simulink model "hydrofoil_sim_unified"  (R2024b)
settings: Solver=VariableStepAuto  StartTime=0.0  StopTime=20  FixedStep=0.05  MaxStep=0.2  RelTol=1e-3
values from neighbouring files (symbols this model uses):
  AfoilA = 0.046    [model_parameters.m]
  AfoilFP = 0.048    [model_parameters.m]
  AfoilFS = 0.048    [model_parameters.m]
  alpha0012 = data0012(:,1)    [model_parameters.m]
  alpha63412wing = data63412wing(:,1)    [model_parameters.m]
  cd0012 = data0012(:,3)    [model_parameters.m]
  cdi63412wing = data63412wing(:,4)    [model_parameters.m]
  cdv63412wing = data63412wing(:,5)    [model_parameters.m]
  cl63412wing = data63412wing(:,3)    [model_parameters.m]
  cm63412wing = data63412wing(:,9)    [model_parameters.m]
  csA = 0.1    [model_parameters.m]
  csF = 0.08    [model_parameters.m]
  deltat = 1/100    (= 0.01)    [model_parameters.m]
  foilA_ARM = [-dxa, dya, dza]    [model_parameters.m]
  foilFP_ARM = [dxf, -dyf, dzf]    [model_parameters.m]
  foilFS_ARM = [dxf, dyf, dzf]    [model_parameters.m]
  g = 9.81    [model_parameters.m]
  LAd = 0.08*pi*(0.8)^3/64    (= 0.0020106192983)    [model_parameters.m]
  LFPd = integral(fpint, foilFP_ARM(2)-0.4, foilFP_ARM(2)+0.4)    [model_parameters.m]
  LFSd = integral(fsint, foilFS_ARM(2)-0.4, foilFS_ARM(2)+0.4)    [model_parameters.m]
  M_RB_1 = inv(M_RB)    [dimensionalize_model.m]    (also in model_parameters.m = M_RB^(-1))
  MAC_A = 0.08    [model_parameters.m]
  MAC_FP = 0.08    [model_parameters.m]
  MAC_FS = 0.08    [model_parameters.m]
  mass = 215    [dimensionalize_model.m]    (also in model_parameters.m)
  propwake = 0.05    [model_parameters.m]
  psd_acc = (9.81*60*1e-6)^2    (= 3.4644996e-07)    [model_parameters.m]
  psd_gyro = (1.222*1e-4)^2    (= 1.493284e-08)    [model_parameters.m]
  r_g = [0; 0; 0]    [dimensionalize_model.m]    (also in model_parameters.m = [xg, yg, zg])
  rho = 1024.8    [model_parameters.m]
  seed_accX = 1324    [model_parameters.m]
  seed_accZ = 1432    [model_parameters.m]
  seed_gps = 4321    [model_parameters.m]
  seed_gyroX = 243251    [model_parameters.m]
  seed_gyroY = 3124234    [model_parameters.m]
  seed_pitch = 7568    [model_parameters.m]
  seed_roll = 35642    [model_parameters.m]
  seed_sonar = 1234    [model_parameters.m]
  setpoint_signals = setpoints.preview    [model_parameters.m]
  sonar_position = [dxf+0.5; 0; -0.1]    [model_parameters.m]
  spanA = 0.76    [model_parameters.m]
  spanFP = 0.76    [model_parameters.m]
  spanFS = 0.76    [model_parameters.m]
  tA = 0.12*0.08    (= 0.0096)    [model_parameters.m]
  tFP = 0.12*0.08    (= 0.0096)    [model_parameters.m]
  tFS = 0.12*0.08    (= 0.0096)    [model_parameters.m]
  usted = 7    [model_parameters.m]
  var_angle = deg2rad(0.2)^2    [model_parameters.m]
  var_gps = 0.05^2    (= 0.0025)    [model_parameters.m]
  var_sonar = 0.002^2    (= 4e-06)    [model_parameters.m]
  wagC1 = 0.165    [model_parameters.m]
  wagC2 = 0.335    [model_parameters.m]
  wage1 = 0.0455*(usted/(MAC_FP/2))    (= 7.9625)    [model_parameters.m]
  wage2 = 0.3*(usted/(MAC_FP/2))    (= 52.5)    [model_parameters.m]
  wave_data = struct('amplitude',0,'omega',0,'wavenumber',0,'phase',0,'direction',0)    [model_parameters.m]
  zpr = dza    (= 0.96)    [model_parameters.m]
undefined symbols (not defined in the file or in its folder): act_lims, actuation_tau, bA, bB, bC, bD, dLTI_array_IDP, dLTI_array_IP, Ka, Klqid, magnitude, PredictionHorizon, set, Ts_reference_preview, V_vals
libraries: mssSimulink x15, mpclib x10, simulink x6, simulink_extras x5, cstblocks x4, matrix_library x3, slpidlib x1
(part 1 of 3)
settings Model: SimulationMode=accelerator  PauseTimes=0.5  SnapshotInterval=1  Creator=jskounakis  LastModifiedBy=jskounakis
settings DataIOCC: ExternalInput=setpoint_reference  InitialState=getstatestruct(report6)
settings OptimizationCC: ReuseModelBlockBuffer=off
settings RTWCC: GPUComputeCapability=3.5

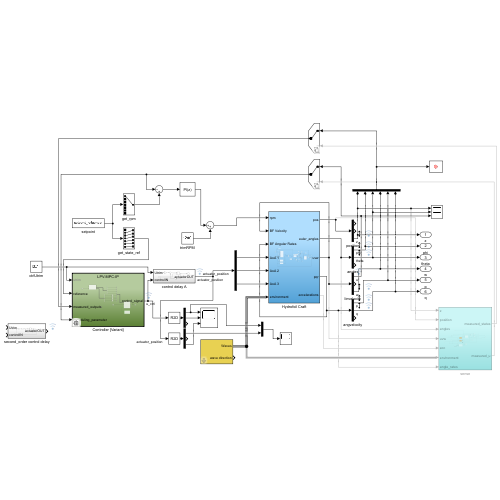
[thumbnail: Simulink's stored preview of the top-level diagram]
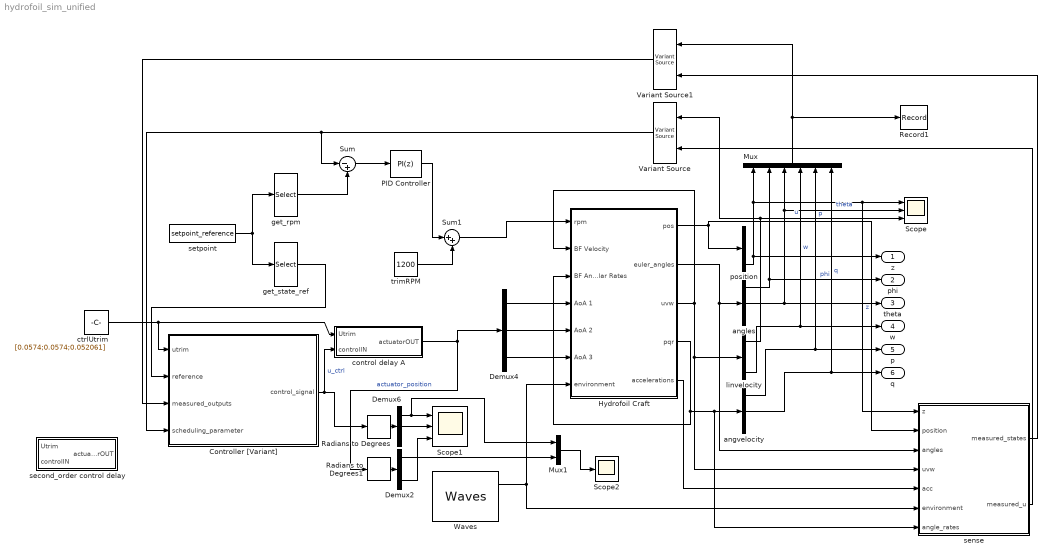
== system hydrofoil_sim_unified ==
  Controller [Variant] : Subsystem  Variant=on  VariantActivationTime=startup
  Demux2 : Demux  Outputs=3
  Demux4 : Demux  Outputs=3
  Demux6 : Demux  Outputs=3
  Hydrofoil Craft : Subsystem
  Mux : Mux  Inputs=6
  Mux1 : Mux  Inputs=2
  PID Controller : slpidlib/PID Controller  Controller=PI  Form=Parallel  TimeDomain=Discrete-time  UseExternalTs=off  SampleTime=1/100  IntegratorMethod=Forward Euler  FilterMethod=Forward Euler  ControllerParametersSource=internal  P=250  I=200  UseKiTs=off  D=0  UseExternalDerivativeSource=off  N=100  UseFilter=on  TunerSelectOption=Transfer Function Based (PID Tuner App)  InitialConditionSource=internal  InitialConditionForIntegrator=0  InitialConditionForFilter=0  DifferentiatorICPrevScaledInput=0  ExternalReset=none  TrackingMode=off  Kt=1  LimitOutput=off  SatLimitsSource=internal  UpperSaturationLimit=inf  LowerSaturationLimit=-inf  LinearizeAsGain=on  AntiWindupMode=none  Kb=1  LimitIntegrator=off  UpperIntegratorSaturationLimit=inf  LowerIntegratorSaturationLimit=-inf  POutMin=[]  POutMax=[]  IOutMin=[]  IOutMax=[]  DOutMin=[]  DOutMax=[]  NOutMin=[]  NOutMax=[]  SumOutMin=[]  SumOutMax=[]  SaturationOutMin=[]  SaturationOutMax=[]  PParamMin=[]  PParamMax=[]  IParamMin=[]  IParamMax=[]  DParamMin=[]  DParamMax=[]  NParamMin=[]  NParamMax=[]  KbParamMin=[]  KbParamMax=[]  KtParamMin=[]  KtParamMax=[]  KbOutMin=[]  KbOutMax=[]  KtOutMin=[]  KtOutMax=[]  IntegratorOutMin=[]  IntegratorOutMax=[]  FilterOutMin=[]  FilterOutMax=[]  SumI1OutMin=[]  SumI1OutMax=[]  SumI2OutMin=[]  SumI2OutMax=[]  SumI3OutMin=[]  SumI3OutMax=[]  SumI4OutMin=[]  SumI4OutMax=[]  SumDOutMin=[]  SumDOutMax=[]  DifferentiatorOutMin=[]  DifferentiatorOutMax=[]  FilterDiffOutCoefMin=[]  FilterDiffOutCoefMax=[]  ReciprocalOutMin=[]  ReciprocalOutMax=[]  SumDenOutMin=[]  SumDenOutMax=[]  SumNumOutMin=[]  SumNumOutMax=[]  DivideOutMin=[]  DivideOutMax=[]  UdiffTsProdOutMin=[]  UdiffTsProdOutMax=[]  NTsProdOutMin=[]  NTsProdOutMax=[]  UintegralTsProdOutMin=[]  UintegralTsProdOutMax=[]  UngainTsProdOutMin=[]  UngainTsProdOutMax=[]  ClampingZeroOutDataTypeStr=Inherit: Inherit via back propagation  ClampingZeroOutMin=[]  ClampingZeroOutMax=[]  FilterDenConstantOutDataTypeStr=Inherit: Inherit via back propagation  FilterDenConstantOutMin=[]  FilterDenConstantOutMax=[]  PCopyOutDataTypeStr=Inherit: Inherit via back propagation  PCopyOutMin=[]  PCopyOutMax=[]  NCopyOutDataTypeStr=Inherit: Inherit via back propagation  NCopyOutMin=[]  NCopyOutMax=[]  IntegratorContinuousStateAttributes=''  IntegratorStateMustResolveToSignalObject=off  IntegratorRTWStateStorageClass=Auto  FilterContinuousStateAttributes=''  FilterStateMustResolveToSignalObject=off  FilterRTWStateStorageClass=Auto  ParallelPVariant=InternalParameters  IdealPVariant=Disabled  IVariant=InternalParameters  DVariant=Disabled  IntegratorVariant=Discrete  SatVariant=Disabled  AWVariant=Passthrough  PCopyVariant=Disabled  TRVariant=Disabled  FdbkBlocksVariant=Forward  IdealPFdbkVariant=Disabled  SatFdbkVariant=Disabled  DerivativeFilterVariant=Disabled  NVariant=Disabled  NCopyVariant=Disabled_SignalSpec  FilterICVariant=Disabled  IntegratorICVariant=InternalICs  ExternalResetVariant=Disabled  TRSumVariant=Passthrough  SumFdbkVariant=Disabled  SumVariant=Sum_PI  TsampFilterVariant=InternalTs  TsampNgainVariant=Passthrough  TsampIntegralVariant=Disabled_SignalSpec  ExternalSaturationOutDataTypeStr=Inherit: Same as second input  DerivativeSourceVariant=Disabled  PreIntVariant=InternalPreInt
  Radians to Degrees : simulink_extras/Transformations/Radians to Degrees
  Radians to Degrees1 : simulink_extras/Transformations/Radians to Degrees
  Record1 : Record  FileSettingsInternal="{\"entries\":[{\"content\":{\"excelSettings\":{\"content\":{},\"type\":\"Streamout.ExcelSettings\"}},\"type\":\"Streamout.FileSettingStorage\",\"uuid\":\"\"}],\"packageUris\":[\"http:\\/\\/schema.mathworks.com\\/mf0\\/streamout_blocks\\/R2020a\"],\"version\":\"1.0\"}"  Layout=[1 1]  SignalsInternal="{\"entries\":[{\"content\":{\"signals\":[{\"content\":{\"blockPath\":[],\"dimensions\":[6],\"domain\":\"\",\"hasChildren\":true,\"lineColor\":\"#7e2f8e\",\"lineWidth\":2,\"port\":1,\"sid\":[\"\"],\"signalID\":1,\"signalName\":\"Mux\"},\"type\":\"RecordBlkView.Signal\",\"uuid\":\"\"},{\"content\":{\"blockPath\":[],\"channel\":[1],\"dimensions\":[6],\"domain\":\"\",\"lineColor\":\"#ff6929\",\"lineWidth\":2,\"parentID\":1,\"plots\":[ 1, 27 ],\"port\":1,\"sid\":[\"\"],\"signalID\":2,\"signalName\":\"Mux\"},\"type\":\"RecordBlkView.Signal\",\"uuid\":\"\"},{\"content\":{\"blockPath\":[],\"channel\":[2],\"dimensions\":[6],\"domain\":\"\",\"lineColor\":\"#b746ff\",\"lineWidth\":2,\"parentID\":1,\"plots\":[ 1 ],\"port\":1,\"sid\":[\"\"],\"signalID\":3,\"signalName\":\"Mux\"},\"type\":\"RecordBlkView.Signal\",\"uuid\":\"\"},{\"content\":{\"blockPath\":[],\"channel\":[3],\"dimensions\":[6],\"domain\":\"\",\"lineColor\":\"#64d413\",\"lineWidth\":2,\"parentID\":1,\"plots\":[ 1, 27 ],\"port\":1,\"sid\":[\"\"],\"signalID\":4,\"signalName\":\"Mux\"},\"type\":\"RecordBlkView.Signal\",\"uuid\":\"\"},{\"content\":{\"blockPath\":[],\"channel\":[4],\"dimensions\":[6],\"domain\":\"\",\"lineColor\":\"#ff13a6\",\"lineWidth\":2,\"parentID\":1,\"plots\":[ 1 ],\"port\":1,\"sid\":[\"\"],\"signalID\":5,\"signalName\":\"Mux\"},\"type\":\"RecordBlkView.Signal\",\"uuid\":\"\"},{\"content\":{\"blockPath\":[],\"channel\":[5],\"dimensions\":[6],\"domain\":\"\",\"lineColor\":\"#ff6929\",\"lineWidth\":2,\"parentID\":1,\"plots\":[ 1 ],\"port\":1,\"sid\":[\"\"],\"signalID\":6,\"signalName\":\"Mux\"},\"type\":\"RecordBlkView.Signal\",\"uuid\":\"\"},{\"content\":{\"blockPath\":[],\"channel\":[6],\"dimensions\":[6],\"domain\":\"\",\"lineColor\":\"#139fff\",\"lineWidth\":2,\"parentID\":1,\"plots\":[ 1 ],\"port\":1,\"sid\":[\"\"],\"signalID\":7,\"signalName\":\"Mux\"},\"type\":\"RecordBlkView.Signal\",\"uuid\":\"\"}]},\"type\":\"RecordBlkView.InputSignals\",\"uuid\":\"\"}],\"packageUris\":[\"http:\\/\\/schema.mathworks.com\\/mf0\\/streamout_blocks\\/R2020a\"],\"version\":\"1.0\"}"  VisualizationBindings="{\"sparklinesplugin\":{\"info\":[{\"bindingParametersList\":[],\"subplotID\":1}]}}"
  Scope : Scope  NumInputPorts=3
  Scope1 : Scope  NumInputPorts=3
  Scope2 : Scope
  Sum : Sum  Inputs=|-+
  Sum1 : Sum  Inputs=|++
  Variant Source : VariantSource
  Variant Source1 : VariantSource
  Waves : mssSimulink/Environment/Waves/Waves  spectrum_type=Predefined waves  disp_flag=off  plot_spectrum=off  plot_realization=off  hs=0.4  omega_peak=6  psi_mean=pi  gamma=3.3  spread=3  depth=inf  nfreq=40  ndir=10  energylim=40  freq_cutoff=2  dir_cutoff=pi/8  rand_seed=seed_waves  rand_freq=on  rand_dir=on  Zeta_a=wave_data.amplitude  Omega=wave_data.omega  Phase=wave_data.phase  Wavenum=wave_data.wavenumber  Psi=wave_data.direction
  angles : Demux  Outputs=3
  angvelocity : Demux  Outputs=3
  control delay A : Subsystem
  ctrlUtrim : Constant  Value=[0.0574;0.0574;0.052061]
  get_rpm : Selector  InputPortWidth=7  IndexOptions=Index vector (dialog)  Indices=[1]  OutputSizes=1
  get_state_ref : Selector  InputPortWidth=7  IndexOptions=Index vector (dialog)  Indices=[2:7]  OutputSizes=1
  linvelocity : Demux  Outputs=3
  position : Demux  Outputs=3
  second_order control delay : Subsystem
  sense : Subsystem
  setpoint : FromWorkspace  VariableName=setpoint_reference
  trimRPM : Constant  Value=1200
  z : Outport
  phi : Outport  Port=2
  theta : Outport  Port=3
  w : Outport  Port=4
  p : Outport  Port=5
  q : Outport  Port=6
  wires:
  ctrlUtrim/1 -> control delay A/1(Utrim), Controller [Variant]/1(utrim)
  Demux4/1 -> Hydrofoil Craft/4(AoA 1)
  Demux4/2 -> Hydrofoil Craft/5(AoA 2)
  Controller [Variant]/1(control_signal) -> control delay A/2(controlIN), Radians to Degrees/1  "u_ctrl"
  angvelocity/2 -> Mux/6, q/1  "q"
  Hydrofoil Craft/4(pqr) -> angvelocity/1, sense/7(angle_rates), Hydrofoil Craft/3(BF Angular Rates)
  Mux/1 -> Variant Source1/1, Record1/1
  angvelocity/1 -> Mux/5, p/1  "p"
  Hydrofoil Craft/3(uvw) -> sense/4(uvw), linvelocity/1, Hydrofoil Craft/2(BF Velocity)
  Hydrofoil Craft/2(euler_angles) -> sense/3(angles), angles/1
  linvelocity/3 -> Mux/4, w/1  "w"
  angles/1 -> Mux/2, phi/1  "phi"
  Hydrofoil Craft/1(pos) -> position/1, sense/2(position)
  angles/2 -> theta/1, Mux/3, Scope/2  "theta"
  position/3 -> Mux/1, Scope/1, sense/1(z), z/1  "z"
  Demux4/3 -> Hydrofoil Craft/6(AoA 3)
  linvelocity/1 -> Variant Source/1, Scope/3  "u"
  Radians to Degrees/1 -> Demux6/1
  Radians to Degrees1/1 -> Demux2/1
  setpoint/1 -> get_rpm/1, get_state_ref/1
  get_state_ref/1 -> Controller [Variant]/2(reference)
  Waves/1 -> sense/6(environment), Hydrofoil Craft/7(environment)
  Demux6/1 -> Mux1/1, Scope1/1
  Demux6/2 -> Scope1/2
  Hydrofoil Craft/5(accelerations) -> sense/5(acc)
  sense/1(measured_states) -> Variant Source1/2
  sense/2(measured_u) -> Variant Source/2
  Variant Source1/1 -> Controller [Variant]/3(measured_outputs)
  Variant Source/1 -> Sum/1, Controller [Variant]/4(scheduling_parameter)
  Mux1/1 -> Scope2/1
  Demux2/1 -> Mux1/2
  control delay A/1(actuatorOUT) -> Demux4/1, Radians to Degrees1/1  "actuator_position"
  Demux2/3 -> Scope1/3
  Sum/1 -> PID Controller/1
  trimRPM/1 -> Sum1/2
  PID Controller/1 -> Sum1/1
  get_rpm/1 -> Sum/2
  Sum1/1 -> Hydrofoil Craft/1(rpm)

== system hydrofoil_sim_unified/Controller [Variant] ==
  note: LPV-MPC
  note: MPC
  note: LQI
  note: 1) Add Subsystem or Model blocks as valid variant choices.
      | 2) You cannot connect blocks at this level. At simulation, connectivity is automatically
      | determined, based on the active variant and port name matching.
  utrim : Inport
  reference : Inport  Port=2
  measured_outputs : Inport  Port=3
  scheduling_parameter : Inport  Port=4
  LPV-MPC-IDP : Subsystem  TreatAsAtomicUnit=on  VariantControl=control_flag == 12
  LPV-MPC-IP : Subsystem  TreatAsAtomicUnit=on  VariantControl=control_flag == 11
  LQI : Subsystem  TreatAsAtomicUnit=on  VariantControl=control_flag == 1
  LQI-S : Subsystem  TreatAsAtomicUnit=on  VariantControl=control_flag == 2
  LQI-SW : Subsystem  TreatAsAtomicUnit=on  VariantControl=control_flag == 3
  MPC : Subsystem  TreatAsAtomicUnit=on  VariantControl=control_flag == 4
  MPC-I : Subsystem  TreatAsAtomicUnit=on  VariantControl=control_flag == 5
  MPC-ID : Subsystem  TreatAsAtomicUnit=on  VariantControl=control_flag == 8
  MPC-IDP : Subsystem  TreatAsAtomicUnit=on  VariantControl=control_flag == 10
  MPC-IO : Subsystem  TreatAsAtomicUnit=on  VariantControl=control_flag == 7
  MPC-IOP : Subsystem  TreatAsAtomicUnit=on  VariantControl=control_flag == 13
  MPC-IP : Subsystem  TreatAsAtomicUnit=on  VariantControl=control_flag == 9
  MPC-O : Subsystem  TreatAsAtomicUnit=on  VariantControl=control_flag == 6
  control_signal : Outport

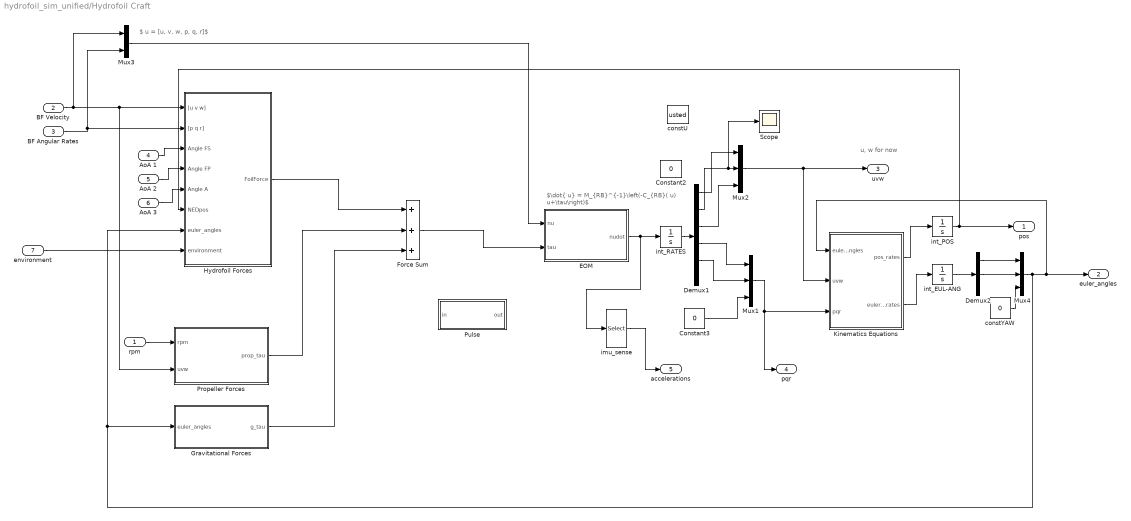
== system hydrofoil_sim_unified/Hydrofoil Craft ==
  note: $\nu = [u, v, w, p, q, r]$
  note: $\dot{\nu} = M_{RB}^{-1}\left(-C_{RB}(\nu)\nu+\tau\right)$
  note: u, w for now
  rpm : Inport
  BF Velocity : Inport  Port=2
  BF Angular Rates : Inport  Port=3
  AoA 1 : Inport  Port=4
  AoA 2 : Inport  Port=5
  AoA 3 : Inport  Port=6
  environment : Inport  Port=7
  Constant2 : Constant  Value=0
  Constant3 : Constant  Value=0
  Demux1 : Demux  Outputs=6
  Demux2 : Demux  Outputs=3
  EOM : Subsystem
  Force Sum : Sum  Inputs=+++
  Gravitational Forces : MATLAB Function  TreatAsAtomicUnit=on
  Hydrofoil Forces : Subsystem
  Kinematics Equations : MATLAB Function  TreatAsAtomicUnit=on
  Mux1 : Mux  Inputs=3
  Mux2 : Mux  Inputs=3
  Mux3 : Mux  Inputs=2
  Mux4 : Mux  Inputs=3
  Propeller Forces : Subsystem
  Pulse : Subsystem
  Scope : Scope
  constU : Constant  Value=usted
  constYAW : Constant  Value=0
  imu_sense : Selector  InputPortWidth=6  IndexOptions=Index vector (dialog)  Indices=[1:3]  OutputSizes=1
  int_EUL-ANG : Integrator  InitialCondition=[0;0;0]
  int_POS : Integrator  InitialCondition=[0;0;-0.3]
  int_RATES : Integrator  InitialCondition=[7;0;0;0;0;0]
  pos : Outport
  euler_angles : Outport  Port=2
  uvw : Outport  Port=3
  pqr : Outport  Port=4
  accelerations : Outport  Port=5
  wires:
  BF Angular Rates/1 -> Mux3/2, Hydrofoil Forces/2("[p q r]")
  BF Velocity/1 -> Mux3/1, Propeller Forces/2(uvw), Hydrofoil Forces/1("[u v w]")
  int_RATES/1 -> Demux1/1
  Mux1/1 -> Kinematics Equations/3(pqr), pqr/1
  Demux1/3 -> Mux2/3
  Demux1/5 -> Mux1/2
  Mux2/1 -> Kinematics Equations/2(uvw), uvw/1
  Kinematics Equations/1(pos_rates) -> int_POS/1
  AoA 2/1 -> Hydrofoil Forces/4(Angle FP)
  AoA 3/1 -> Hydrofoil Forces/5(Angle A)
  AoA 1/1 -> Hydrofoil Forces/3(Angle FS)
  Demux2/1 -> Mux4/1
  Demux2/2 -> Mux4/2
  Mux4/1 -> Hydrofoil Forces/7(euler_angles), Gravitational Forces/1(euler_angles), Kinematics Equations/1(euler_angles), euler_angles/1
  constYAW/1 -> Mux4/3
  int_EUL-ANG/1 -> Demux2/1
  rpm/1 -> Propeller Forces/1(rpm)
  Mux3/1 -> EOM/1(nu)
  EOM/1(nudot) -> imu_sense/1, int_RATES/1
  Kinematics Equations/2(euler_ang_rates) -> int_EUL-ANG/1
  Demux1/4 -> Mux1/1
  Constant3/1 -> Mux1/3
  int_POS/1 -> pos/1, Hydrofoil Forces/6(NEDpos)
  Demux1/1 -> Mux2/1
  imu_sense/1 -> accelerations/1
  environment/1 -> Hydrofoil Forces/8(environment)
  Gravitational Forces/1(g_tau) -> Force Sum/3
  Propeller Forces/1(prop_tau) -> Force Sum/2
  Hydrofoil Forces/1(FoilForce) -> Force Sum/1
  Demux1/2 -> Scope/1, Mux2/2
  Force Sum/1 -> EOM/2(tau)

== system hydrofoil_sim_unified/control delay A ==
  Utrim : Inport
  controlIN : Inport  Port=2
  Integrator : Integrator  InitialConditionSource=external
  Sum2 : Sum  Inputs=|+-
  delayU : Gain  Gain=actuation_tau
  delayUc : Gain  Gain=actuation_tau
  actuatorOUT : Outport
  wires:
  delayU/1 -> Sum2/2
  delayUc/1 -> Sum2/1
  Integrator/1 -> actuatorOUT/1, delayU/1
  Sum2/1 -> Integrator/1
  controlIN/1 -> delayUc/1
  Utrim/1 -> Integrator/2

== system hydrofoil_sim_unified/second_order control delay ==
  Utrim : Inport
  controlIN : Inport  Port=2
  1/J : Gain  Gain=1/0.04
  Integrator : Integrator  InitialConditionSource=external
  Integrator1 : Integrator
  Saturation : Saturate
  Sum1 : Sum  Inputs=|+-
  Sum2 : Sum  Inputs=|+-
  b : Gain  Gain=0.7
  p : Gain  Gain=15
  actuatorOUT : Outport
  wires:
  Sum1/1 -> 1/J/1
  controlIN/1 -> Sum2/1
  1/J/1 -> Integrator1/1
  p/1 -> Saturation/1
  Utrim/1 -> Integrator/2
  Integrator/1 -> actuatorOUT/1, Sum2/2
  Saturation/1 -> Sum1/1
  b/1 -> Sum1/2
  Sum2/1 -> p/1
  Integrator1/1 -> Integrator/1, b/1

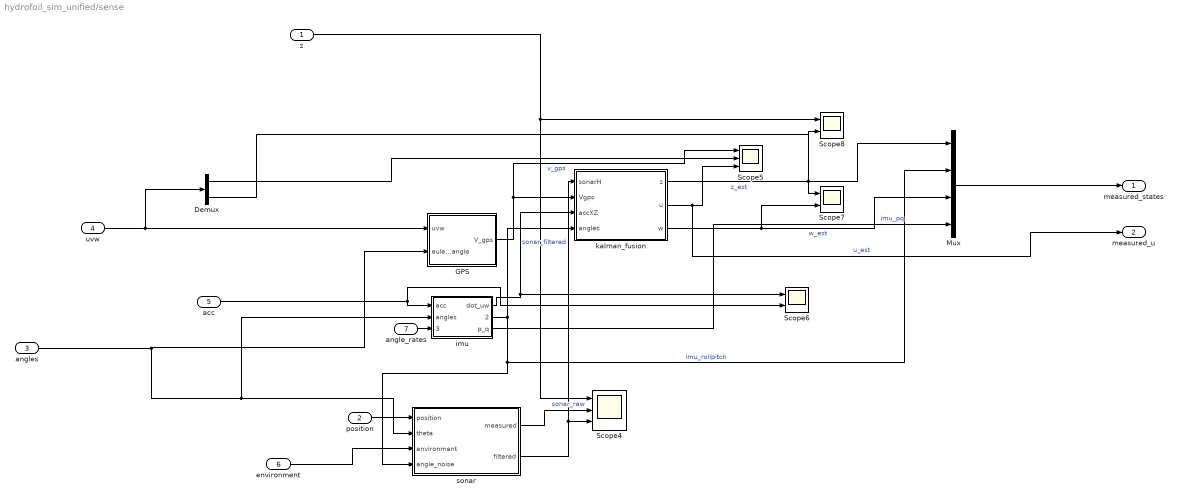
== system hydrofoil_sim_unified/sense ==
  z : Inport
  position : Inport  Port=2
  angles : Inport  Port=3
  uvw : Inport  Port=4
  acc : Inport  Port=5
  environment : Inport  Port=6
  angle_rates : Inport  Port=7
  Demux : Demux  Outputs=3
  GPS : Subsystem  TreatAsAtomicUnit=on
  Mux : Mux
  Scope4 : Scope  NumInputPorts=3
  Scope5 : Scope  NumInputPorts=3
  Scope6 : Scope  NumInputPorts=2
  Scope7 : Scope  NumInputPorts=2
  Scope8 : Scope  NumInputPorts=2
  imu : Subsystem
  kalman_fusion : MATLAB Function  TreatAsAtomicUnit=on  SystemSampleTime=deltat
  sonar : Subsystem
  measured_states : Outport
  measured_u : Outport  Port=2
  wires:
  imu/1(dot_uw) -> kalman_fusion/3(accXZ), Scope6/1
  GPS/1(V_gps) -> Scope5/1, kalman_fusion/2(Vgps)  "v_gps"
  kalman_fusion/3(w) -> Mux/3, Scope7/2  "w_est"
  kalman_fusion/2(u) -> measured_u/1, Scope5/3  "u_est"
  sonar/1(measured) -> Scope4/2  "sonar_raw"
  kalman_fusion/1(z) -> Mux/1, Scope8/2  "z_est"
  acc/1 -> Scope6/2, imu/1(acc)
  angles/1 -> imu/2(angles), sonar/2(theta), GPS/2(euler_angle)
  sonar/2(filtered) -> kalman_fusion/1(sonarH), Scope4/3  "sonar_filtered"
  angle_rates/1 -> imu/3(angle_rates)
  position/1 -> sonar/1(position)
  z/1 -> Scope8/1, Scope4/1
  uvw/1 -> Demux/1, GPS/1(uvw)
  environment/1 -> sonar/3(environment)
  Demux/3 -> Scope7/1
  Demux/1 -> Scope5/2
  imu/2(roll_pitch) -> Mux/2, sonar/4(angle_noise), kalman_fusion/4(angles)  "imu_rollpitch"
  imu/3(p_q) -> Mux/4  "imu_pq"
  Mux/1 -> measured_states/1

== system hydrofoil_sim_unified/Controller [Variant]/LPV-MPC-IDP ==
  reference : Inport
  measured_outputs : Inport  Port=2
  scheduling_parameter : Inport  Port=3
  Adaptive MPC Controller : mpclib/Adaptive MPC Controller  SCDEnableBlockLinearizationSpecification=on  mpcobj=lpv_mpc_IDP  enable_value=0  updateMPCinCallerWorkspace=on  md_inport=off  mv_inport=off  uref_inport=off  return_cost=off  return_mvseq=on  return_qpstatus=off  return_xseq=off  return_state=off  return_ovseq=on  state_inport=off  isltv_plant=off  umin_inport=off  umax_inport=off  ymin_inport=off  ymax_inport=off  cc_inport=off  ywt_inport=off  uwt_inport=off  duwt_inport=off  rhoeps_inport=off  pm_inport=off  MaximumP=10  HorizonChoice=FixedHorizon  BlockDataType=double  SampleTimeInherited=off  switch_inport=off
  Bus Creator : BusCreator  Inputs=8
  Bus Selector : BusSelector  OutputSignals=A,B,C,D
  Bus Selector2 : BusSelector  OutputSignals=InputOffset,OutputOffset,StateOffset,StateUpdateOffset
  Gain : Gain
  Gain1 : Gain
  Gain2 : Gain
  Gain3 : Gain  Gain=0
  LPV System : cstblocks/Linear Parameter Varying/LPV System  sys=set(dLTI_array_IDP, 'SamplingGrid', struct('V', V_vals));  InitialConditionSource=internal  InitialCondition=0  opSpecOption=Specify offsets as double arrays  uOffset=U_offset  yOffset=Y_offset  xOffset=[0;0;0;0;0;0;0;0;0]  opEquilOption=on  dxOffset=0  AFixed=false  BFixed=false  CFixed=false  DFixed=false  uDelayFixed=false  yDelayFixed=false  iDelayFixed=false  sysFixedOption=First model in state-space array  sysFixed=[]  IMethod=Linear  EMethod=Clip  IndexSearch=Binary search  IndexBegin=on  OutputX=on  OutputXdot=off  OutputLTI=on  OutputOP=on  DataType=double  InitBufferSize=1024  FixedBuffer=off  SimMode=Interpreted execution  Offset=struct
  Reference Previewer : Subsystem  mask{signal=setpoint_signals, ts=Ts_reference_preview, steps=PredictionHorizon}
      mask prompts: signal "Signal name"; ts "Sampling time"; steps "Number of previewing steps"
      mask init:
      | ts = evalin('base',get_param(gcbh,'ts'));
      | signal = evalin('base',get_param(gcbh,'signal'));
      | steps = evalin('base',get_param(gcbh,'steps'));
      | data = mpc_previewer_maskinit(signal,ts);
      mask Display:
      | fprintf('Future\nsample\nextractor');
      | port_label('output', 1, 'seq')
      | port_label('output', 2, '@t')
  control_signal : Outport
  wires:
  Gain1/1 -> Bus Creator/6  "Y"
  Bus Selector2/1 -> Gain/1  "<InputOffset>"
  Bus Selector2/3 -> Gain2/1  "<StateOffset>"
  Bus Selector/2 -> Bus Creator/2  "<B>"
  LPV System/4 -> Bus Selector2/1
  Bus Selector/4 -> Bus Creator/4  "<D>"
  Bus Selector2/4 -> Gain3/1  "<StateUpdateOffset>"
  Gain3/1 -> Bus Creator/8  "DX"
  Gain2/1 -> Bus Creator/7  "X"
  measured_outputs/1 -> Adaptive MPC Controller/2
  Bus Selector/3 -> Bus Creator/3  "<C>"
  Bus Creator/1 -> Adaptive MPC Controller/1
  Bus Selector/1 -> Bus Creator/1  "<A>"
  scheduling_parameter/1 -> LPV System/2
  Gain/1 -> Bus Creator/5  "U"
  Bus Selector2/2 -> Gain1/1  "<OutputOffset>"
  Adaptive MPC Controller/1 -> control_signal/1
  LPV System/3 -> Bus Selector/1
  Reference Previewer/1(sequence) -> Adaptive MPC Controller/3

== system hydrofoil_sim_unified/Controller [Variant]/LPV-MPC-IP ==
  reference : Inport
  measured_outputs : Inport  Port=2
  scheduling_parameter : Inport  Port=3
  Adaptive MPC Controller : mpclib/Adaptive MPC Controller  SCDEnableBlockLinearizationSpecification=on  mpcobj=lpv_mpc_IP  enable_value=0  updateMPCinCallerWorkspace=on  md_inport=off  mv_inport=off  uref_inport=off  return_cost=off  return_mvseq=on  return_qpstatus=off  return_xseq=off  return_state=off  return_ovseq=on  state_inport=off  isltv_plant=off  umin_inport=off  umax_inport=off  ymin_inport=off  ymax_inport=off  cc_inport=off  ywt_inport=off  uwt_inport=off  duwt_inport=off  rhoeps_inport=off  pm_inport=off  MaximumP=10  HorizonChoice=FixedHorizon  BlockDataType=double  SampleTimeInherited=off  switch_inport=off
  Bus Creator : BusCreator  Inputs=8
  Bus Selector : BusSelector  OutputSignals=A,B,C,D
  Bus Selector2 : BusSelector  OutputSignals=InputOffset,OutputOffset,StateOffset,StateUpdateOffset
  Gain : Gain
  Gain1 : Gain
  Gain2 : Gain
  Gain3 : Gain  Gain=0
  LPV System : cstblocks/Linear Parameter Varying/LPV System  sys=set(dLTI_array_IP, 'SamplingGrid', struct('V', V_vals));  InitialConditionSource=internal  InitialCondition=0  opSpecOption=Specify offsets as double arrays  uOffset=U_offset  yOffset=Y_offset  xOffset=[0;0;0;0;0;0]  opEquilOption=on  dxOffset=0  AFixed=false  BFixed=false  CFixed=false  DFixed=false  uDelayFixed=false  yDelayFixed=false  iDelayFixed=false  sysFixedOption=First model in state-space array  sysFixed=[]  IMethod=Linear  EMethod=Clip  IndexSearch=Binary search  IndexBegin=on  OutputX=on  OutputXdot=off  OutputLTI=on  OutputOP=on  DataType=double  InitBufferSize=1024  FixedBuffer=off  SimMode=Interpreted execution  Offset=struct
  Reference Previewer : Subsystem  mask{signal=setpoint_signals, ts=Ts_reference_preview, steps=PredictionHorizon}
      mask prompts: signal "Signal name"; ts "Sampling time"; steps "Number of previewing steps"
      mask init:
      | ts = evalin('base',get_param(gcbh,'ts'));
      | signal = evalin('base',get_param(gcbh,'signal'));
      | steps = evalin('base',get_param(gcbh,'steps'));
      | data = mpc_previewer_maskinit(signal,ts);
      mask Display:
      | fprintf('Future\nsample\nextractor');
      | port_label('output', 1, 'seq')
      | port_label('output', 2, '@t')
  control_signal : Outport
  wires:
  Gain1/1 -> Bus Creator/6  "Y"
  Bus Selector2/1 -> Gain/1  "<InputOffset>"
  Bus Selector2/3 -> Gain2/1  "<StateOffset>"
  Bus Selector/2 -> Bus Creator/2  "<B>"
  LPV System/4 -> Bus Selector2/1
  Bus Selector/4 -> Bus Creator/4  "<D>"
  Bus Selector2/4 -> Gain3/1  "<StateUpdateOffset>"
  Gain3/1 -> Bus Creator/8  "DX"
  Gain2/1 -> Bus Creator/7  "X"
  measured_outputs/1 -> Adaptive MPC Controller/2
  Bus Selector/3 -> Bus Creator/3  "<C>"
  Bus Creator/1 -> Adaptive MPC Controller/1
  Bus Selector/1 -> Bus Creator/1  "<A>"
  scheduling_parameter/1 -> LPV System/2
  Gain/1 -> Bus Creator/5  "U"
  Bus Selector2/2 -> Gain1/1  "<OutputOffset>"
  Adaptive MPC Controller/1 -> control_signal/1
  LPV System/3 -> Bus Selector/1
  Reference Previewer/1(sequence) -> Adaptive MPC Controller/3

== system hydrofoil_sim_unified/Controller [Variant]/LQI ==
  utrim : Inport
  reference : Inport  Port=2
  measured_outputs : Inport  Port=3
  Discrete LQRi no S/AW : MATLAB Function  TreatAsAtomicUnit=on  SystemSampleTime=0.1
  control_signal : Outport
  wires:
  reference/1 -> Discrete LQRi no S/AW/1(reference)
  measured_outputs/1 -> Discrete LQRi no S/AW/2(states)
  utrim/1 -> Discrete LQRi no S/AW/3(u_trim)
  Discrete LQRi no S/AW/1(control_input) -> control_signal/1

== system hydrofoil_sim_unified/Controller [Variant]/LQI-S ==
  utrim : Inport
  reference : Inport  Port=2
  measured_outputs : Inport  Port=3
  Discrete LQRi no AW : MATLAB Function  TreatAsAtomicUnit=on  SystemSampleTime=0.1
  control_signal : Outport
  wires:
  reference/1 -> Discrete LQRi no AW/1(reference)
  measured_outputs/1 -> Discrete LQRi no AW/2(states)
  utrim/1 -> Discrete LQRi no AW/3(u_trim)
  Discrete LQRi no AW/1(control_input) -> control_signal/1

== system hydrofoil_sim_unified/Controller [Variant]/LQI-SW ==
  utrim : Inport
  reference : Inport  Port=2
  measured_outputs : Inport  Port=3
  Discrete LQRi : MATLAB Function  TreatAsAtomicUnit=on  SystemSampleTime=0.1
  control_signal : Outport
  wires:
  reference/1 -> Discrete LQRi/1(reference)
  measured_outputs/1 -> Discrete LQRi/2(states)
  utrim/1 -> Discrete LQRi/3(u_trim)
  Discrete LQRi/1(control_input) -> control_signal/1

== system hydrofoil_sim_unified/Controller [Variant]/MPC ==
  reference : Inport
  measured_outputs : Inport  Port=2
  MPC : mpclib/MPC Controller  SCDEnableBlockLinearizationSpecification=on  mpcobj=mpc_base  is_multiple=0  enable_value=0  return_u0=off  updateMPCinCallerWorkspace=on  md_inport=off  mv_inport=off  uref_inport=off  return_cost=off  return_mvseq=on  return_qpstatus=off  return_xseq=off  return_state=off  return_ovseq=on  state_inport=off  umin_inport=off  umax_inport=off  ymin_inport=off  ymax_inport=off  cc_inport=off  ywt_inport=off  uwt_inport=off  duwt_inport=off  rhoeps_inport=off  pm_inport=off  MaximumP=10  HorizonChoice=FixedHorizon  n_ts=0.1  n_p=10  n_mv=3  n_md=0  n_ud=0  n_mo=6  n_uo=0  BlockDataType=double  SampleTimeInherited=off  switch_inport=off
  control_signal : Outport
  wires:
  MPC/1 -> control_signal/1
  measured_outputs/1 -> MPC/1
  reference/1 -> MPC/2

== system hydrofoil_sim_unified/Controller [Variant]/MPC-I ==
  reference : Inport
  measured_outputs : Inport  Port=2
  MPC : mpclib/MPC Controller  SCDEnableBlockLinearizationSpecification=on  mpcobj=mpc_I  is_multiple=0  enable_value=0  return_u0=off  updateMPCinCallerWorkspace=on  md_inport=off  mv_inport=off  uref_inport=off  return_cost=off  return_mvseq=on  return_qpstatus=off  return_xseq=off  return_state=off  return_ovseq=on  state_inport=off  umin_inport=off  umax_inport=off  ymin_inport=off  ymax_inport=off  cc_inport=off  ywt_inport=off  uwt_inport=off  duwt_inport=off  rhoeps_inport=off  pm_inport=off  MaximumP=10  HorizonChoice=FixedHorizon  n_ts=0.1  n_p=10  n_mv=3  n_md=0  n_ud=3  n_mo=6  n_uo=0  BlockDataType=double  SampleTimeInherited=off  switch_inport=off
  control_signal : Outport
  wires:
  MPC/1 -> control_signal/1
  measured_outputs/1 -> MPC/1
  reference/1 -> MPC/2

== system hydrofoil_sim_unified/Controller [Variant]/MPC-ID ==
  reference : Inport
  measured_outputs : Inport  Port=2
  MPC : mpclib/MPC Controller  SCDEnableBlockLinearizationSpecification=on  mpcobj=mpc_ID  is_multiple=0  enable_value=0  return_u0=off  updateMPCinCallerWorkspace=on  md_inport=off  mv_inport=off  uref_inport=off  return_cost=off  return_mvseq=on  return_qpstatus=off  return_xseq=off  return_state=off  return_ovseq=on  state_inport=off  umin_inport=off  umax_inport=off  ymin_inport=off  ymax_inport=off  cc_inport=off  ywt_inport=off  uwt_inport=off  duwt_inport=off  rhoeps_inport=off  pm_inport=off  MaximumP=10  HorizonChoice=FixedHorizon  n_ts=0.1  n_p=10  n_mv=3  n_md=0  n_ud=3  n_mo=6  n_uo=0  BlockDataType=double  SampleTimeInherited=off  switch_inport=off
  control_signal : Outport
  wires:
  MPC/1 -> control_signal/1
  measured_outputs/1 -> MPC/1
  reference/1 -> MPC/2

== system hydrofoil_sim_unified/Controller [Variant]/MPC-IDP ==
  reference : Inport
  measured_outputs : Inport  Port=2
  MPC : mpclib/MPC Controller  SCDEnableBlockLinearizationSpecification=on  mpcobj=mpc_ID  is_multiple=0  enable_value=0  return_u0=off  updateMPCinCallerWorkspace=on  md_inport=off  mv_inport=off  uref_inport=off  return_cost=off  return_mvseq=on  return_qpstatus=off  return_xseq=off  return_state=off  return_ovseq=on  state_inport=off  umin_inport=off  umax_inport=off  ymin_inport=off  ymax_inport=off  cc_inport=off  ywt_inport=off  uwt_inport=off  duwt_inport=off  rhoeps_inport=off  pm_inport=off  MaximumP=10  HorizonChoice=FixedHorizon  n_ts=0.1  n_p=10  n_mv=3  n_md=0  n_ud=3  n_mo=6  n_uo=0  BlockDataType=double  SampleTimeInherited=off  switch_inport=off
  Reference Previewer : Subsystem  mask{signal=setpoint_signals, ts=Ts_reference_preview, steps=PredictionHorizon}
      mask prompts: signal "Signal name"; ts "Sampling time"; steps "Number of previewing steps"
      mask init:
      | ts = evalin('base',get_param(gcbh,'ts'));
      | signal = evalin('base',get_param(gcbh,'signal'));
      | steps = evalin('base',get_param(gcbh,'steps'));
      | data = mpc_previewer_maskinit(signal,ts);
      mask Display:
      | fprintf('Future\nsample\nextractor');
      | port_label('output', 1, 'seq')
      | port_label('output', 2, '@t')
  control_signal : Outport
  wires:
  MPC/1 -> control_signal/1
  measured_outputs/1 -> MPC/1
  Reference Previewer/1(sequence) -> MPC/2

== system hydrofoil_sim_unified/Controller [Variant]/MPC-IO ==
  reference : Inport
  measured_outputs : Inport  Port=2
  MPC : mpclib/MPC Controller  SCDEnableBlockLinearizationSpecification=on  mpcobj=mpc_IO  is_multiple=0  enable_value=0  return_u0=off  updateMPCinCallerWorkspace=on  md_inport=off  mv_inport=off  uref_inport=off  return_cost=off  return_mvseq=on  return_qpstatus=off  return_xseq=off  return_state=off  return_ovseq=on  state_inport=off  umin_inport=off  umax_inport=off  ymin_inport=off  ymax_inport=off  cc_inport=off  ywt_inport=off  uwt_inport=off  duwt_inport=off  rhoeps_inport=off  pm_inport=off  MaximumP=10  HorizonChoice=FixedHorizon  n_ts=0.1  n_p=10  n_mv=3  n_md=0  n_ud=3  n_mo=6  n_uo=0  BlockDataType=double  SampleTimeInherited=off  switch_inport=off
  control_signal : Outport
  wires:
  MPC/1 -> control_signal/1
  measured_outputs/1 -> MPC/1
  reference/1 -> MPC/2

== system hydrofoil_sim_unified/Controller [Variant]/MPC-IOP ==
  measured_outputs : Inport
  MPC : mpclib/MPC Controller  SCDEnableBlockLinearizationSpecification=on  mpcobj=mpc_IO  is_multiple=0  enable_value=0  return_u0=off  updateMPCinCallerWorkspace=on  md_inport=off  mv_inport=off  uref_inport=off  return_cost=off  return_mvseq=on  return_qpstatus=off  return_xseq=off  return_state=off  return_ovseq=on  state_inport=off  umin_inport=off  umax_inport=off  ymin_inport=off  ymax_inport=off  cc_inport=off  ywt_inport=off  uwt_inport=off  duwt_inport=off  rhoeps_inport=off  pm_inport=off  MaximumP=10  HorizonChoice=FixedHorizon  n_ts=0.1  n_p=10  n_mv=3  n_md=0  n_ud=3  n_mo=6  n_uo=0  BlockDataType=double  SampleTimeInherited=off  switch_inport=off
  Reference Previewer : Subsystem  mask{signal=setpoint_signals, ts=Ts_reference_preview, steps=PredictionHorizon}
      mask prompts: signal "Signal name"; ts "Sampling time"; steps "Number of previewing steps"
      mask init:
      | ts = evalin('base',get_param(gcbh,'ts'));
      | signal = evalin('base',get_param(gcbh,'signal'));
      | steps = evalin('base',get_param(gcbh,'steps'));
      | data = mpc_previewer_maskinit(signal,ts);
      mask Display:
      | fprintf('Future\nsample\nextractor');
      | port_label('output', 1, 'seq')
      | port_label('output', 2, '@t')
  control_signal : Outport
  wires:
  MPC/1 -> control_signal/1
  measured_outputs/1 -> MPC/1
  Reference Previewer/1(sequence) -> MPC/2

== system hydrofoil_sim_unified/Controller [Variant]/MPC-IP ==
  measured_outputs : Inport
  MPC : mpclib/MPC Controller  SCDEnableBlockLinearizationSpecification=on  mpcobj=mpc_I  is_multiple=0  enable_value=0  return_u0=off  updateMPCinCallerWorkspace=on  md_inport=off  mv_inport=off  uref_inport=off  return_cost=off  return_mvseq=on  return_qpstatus=off  return_xseq=off  return_state=off  return_ovseq=on  state_inport=off  umin_inport=off  umax_inport=off  ymin_inport=off  ymax_inport=off  cc_inport=off  ywt_inport=off  uwt_inport=off  duwt_inport=off  rhoeps_inport=off  pm_inport=off  MaximumP=10  HorizonChoice=FixedHorizon  n_ts=0.1  n_p=10  n_mv=3  n_md=0  n_ud=3  n_mo=6  n_uo=0  BlockDataType=double  SampleTimeInherited=off  switch_inport=off
  Reference Previewer : Subsystem  mask{signal=setpoint_signals, ts=Ts_reference_preview, steps=PredictionHorizon}
      mask prompts: signal "Signal name"; ts "Sampling time"; steps "Number of previewing steps"
      mask init:
      | ts = evalin('base',get_param(gcbh,'ts'));
      | signal = evalin('base',get_param(gcbh,'signal'));
      | steps = evalin('base',get_param(gcbh,'steps'));
      | data = mpc_previewer_maskinit(signal,ts);
      mask Display:
      | fprintf('Future\nsample\nextractor');
      | port_label('output', 1, 'seq')
      | port_label('output', 2, '@t')
  control_signal : Outport
  wires:
  MPC/1 -> control_signal/1
  measured_outputs/1 -> MPC/1
  Reference Previewer/1(sequence) -> MPC/2

== system hydrofoil_sim_unified/Controller [Variant]/MPC-O ==
  reference : Inport
  measured_outputs : Inport  Port=2
  MPC : mpclib/MPC Controller  SCDEnableBlockLinearizationSpecification=on  mpcobj=mpc_O  is_multiple=0  enable_value=0  return_u0=off  updateMPCinCallerWorkspace=on  md_inport=off  mv_inport=off  uref_inport=off  return_cost=off  return_mvseq=on  return_qpstatus=off  return_xseq=off  return_state=off  return_ovseq=on  state_inport=off  umin_inport=off  umax_inport=off  ymin_inport=off  ymax_inport=off  cc_inport=off  ywt_inport=off  uwt_inport=off  duwt_inport=off  rhoeps_inport=off  pm_inport=off  MaximumP=10  HorizonChoice=FixedHorizon  n_ts=0.1  n_p=10  n_mv=3  n_md=0  n_ud=0  n_mo=6  n_uo=0  BlockDataType=double  SampleTimeInherited=off  switch_inport=off
  control_signal : Outport
  wires:
  MPC/1 -> control_signal/1
  measured_outputs/1 -> MPC/1
  reference/1 -> MPC/2

== system hydrofoil_sim_unified/Hydrofoil Craft/EOM ==
  note: $-C_{RB}(\nu)\nu+\tau$
  note: $M_{RB}^{-1}$
  note: Rigid Body Coriolis - Centripetal Matrix
  note: $M_{RB}^{-1}\left(-C_{RB}(\nu)\nu+\tau\right)$
  nu : Inport
  tau : Inport  Port=2
  Add3 : Sum  Inputs=-+
  CRB MATRIX : MATLAB Function  TreatAsAtomicUnit=on
  MRB INVERSE : Constant  Value=M_RB_1
  Product1 : Product  Multiplication=Matrix(*)
  Product2 : Product  Multiplication=Matrix(*)
  nudot : Outport
  wires:
  CRB MATRIX/1(C) -> Product2/1
  nu/1 -> Product2/2, CRB MATRIX/1(nu)
  Add3/1 -> Product1/2
  Product2/1 -> Add3/1
  tau/1 -> Add3/2
  Product1/1 -> nudot/1
  MRB INVERSE/1 -> Product1/1

== system hydrofoil_sim_unified/Hydrofoil Craft/Hydrofoil Forces ==
  "[u v w]" : Inport
  "[p q r]" : Inport  Port=2
  Angle FS : Inport  Port=3
  Angle FP : Inport  Port=4
  Angle A : Inport  Port=5
  NEDpos : Inport  Port=6
  euler_angles : Inport  Port=7
  environment : Inport  Port=8
  Add : Sum  Inputs=+++
  Hydrofoil [A] : Subsystem
      settings: PortSchema="{\"entries\":[{\"content\":{\"sides\":[{\"content\":{\"connectorIds\":[\"In1\",\"In2\",\"In3\",\"In4\",\"In5\"]},\"type\":\"ConnectorPlacement.EquallySpacedRectSide\",\"uuid\":\"677cb1e4-b507-48e0-bf9b-1d4b68d11740\"},{\"content\":{\"connectorIds\":[\"Out1\"],\"side\":\"RIGHT\"},\"type\":\"ConnectorPlacement.EquallySpacedRectSide\",\"uuid\":\"aaee0231-58d5-427f-802b-fd317cb8babc\"},{\"content\":{\"connectorIds\":[\"In6\"],\"side\":\"TOP\"},\"type\":\"ConnectorPlacement.EquallySpacedRectSide\",\"uuid\":\"1e7dce63-7570-4618-9859-1c6c6aa2cc5b\"}]},\"type\":\"ConnectorPlacement.EquallySpacedConnector\",\"uuid\":\"334cd270-f68d-4b91-93d0-e05f7617c880\"}],\"packageUris\":[\"http://schema.mathworks.com/mf0/Connector/R2020b\"],\"version\":\"1.0\"}"
  Hydrofoil [FP] : Subsystem
      settings: PortSchema="{\"entries\":[{\"content\":{\"sides\":[{\"content\":{\"connectorIds\":[\"In1\",\"In2\",\"In3\",\"In4\",\"In5\"]},\"type\":\"ConnectorPlacement.EquallySpacedRectSide\",\"uuid\":\"677cb1e4-b507-48e0-bf9b-1d4b68d11740\"},{\"content\":{\"connectorIds\":[\"Out1\"],\"side\":\"RIGHT\"},\"type\":\"ConnectorPlacement.EquallySpacedRectSide\",\"uuid\":\"aaee0231-58d5-427f-802b-fd317cb8babc\"},{\"content\":{\"connectorIds\":[\"In6\"],\"side\":\"TOP\"},\"type\":\"ConnectorPlacement.EquallySpacedRectSide\",\"uuid\":\"1e7dce63-7570-4618-9859-1c6c6aa2cc5b\"}]},\"type\":\"ConnectorPlacement.EquallySpacedConnector\",\"uuid\":\"334cd270-f68d-4b91-93d0-e05f7617c880\"}],\"packageUris\":[\"http://schema.mathworks.com/mf0/Connector/R2020b\"],\"version\":\"1.0\"}"
  Hydrofoil [FS] : Subsystem
      settings: PortSchema="{\"entries\":[{\"content\":{\"sides\":[{\"content\":{\"connectorIds\":[\"In1\",\"In2\",\"In3\",\"In4\",\"In5\"]},\"type\":\"ConnectorPlacement.EquallySpacedRectSide\",\"uuid\":\"677cb1e4-b507-48e0-bf9b-1d4b68d11740\"},{\"content\":{\"connectorIds\":[\"Out1\"],\"side\":\"RIGHT\"},\"type\":\"ConnectorPlacement.EquallySpacedRectSide\",\"uuid\":\"aaee0231-58d5-427f-802b-fd317cb8babc\"},{\"content\":{\"connectorIds\":[\"In6\"],\"side\":\"TOP\"},\"type\":\"ConnectorPlacement.EquallySpacedRectSide\",\"uuid\":\"1e7dce63-7570-4618-9859-1c6c6aa2cc5b\"}]},\"type\":\"ConnectorPlacement.EquallySpacedConnector\",\"uuid\":\"334cd270-f68d-4b91-93d0-e05f7617c880\"}],\"packageUris\":[\"http://schema.mathworks.com/mf0/Connector/R2020b\"],\"version\":\"1.0\"}"
  FoilForce : Outport
  wires:
  Angle A/1 -> Hydrofoil [A]/5(Control Deflection (ac))
  Angle FP/1 -> Hydrofoil [FP]/5(Control Deflection (ac))
  "[u v w]"/1 -> Hydrofoil [FS]/1("[u v w]"), Hydrofoil [A]/1("[u v w]"), Hydrofoil [FP]/1("[u v w]")
  "[p q r]"/1 -> Hydrofoil [FP]/2("[p q r]"), Hydrofoil [FS]/2("[p q r]"), Hydrofoil [A]/2("[p q r]")
  Hydrofoil [FP]/1(Force - Moment) -> Add/1
  Add/1 -> FoilForce/1
  euler_angles/1 -> Hydrofoil [FP]/4(euler_angles), Hydrofoil [FS]/4(euler_angles), Hydrofoil [A]/4(euler_angles)
  NEDpos/1 -> Hydrofoil [FP]/3(NEDpos), Hydrofoil [FS]/3(NEDpos), Hydrofoil [A]/3(NEDpos)
  Hydrofoil [A]/1(Force - Moment) -> Add/2
  Angle FS/1 -> Hydrofoil [FS]/5(Control Deflection (ac))
  Hydrofoil [FS]/1(Force - Moment) -> Add/3
  environment/1 -> Hydrofoil [FS]/6(waves), Hydrofoil [A]/6(waves), Hydrofoil [FP]/6(waves)

== system hydrofoil_sim_unified/Hydrofoil Craft/Propeller Forces ==
  rpm : Inport
  uvw : Inport  Port=2
  Gain : Gain  Gain=1/60
  Mux : Mux  Inputs=6
  Open-water propeller characteristics : mssSimulink/Modelling/Propulsion/Open-water propeller characteristics  Par_Thruster_D=propD  Par_Thruster_Ktp=propKtp  Par_Thruster_Kqp=propKqp  Par_Thruster_reverse_reduction=0.8  Glob_rhow=rho
  Product : Product
  Product1 : Product
  Propeller Arm : Constant  Value=zpr
  Selector : Selector  InputPortWidth=3  IndexOptions=Index vector (dialog)  Indices=[1]  OutputSizes=1
  wake : Constant  Value=1-propwake
  prop_tau : Outport
  wires:
  Propeller Arm/1 -> Product/1
  Product/1 -> Mux/5
  wake/1 -> Product1/1
  Product1/1 -> Open-water propeller characteristics/2
  rpm/1 -> Gain/1
  Gain/1 -> Open-water propeller characteristics/1
  Open-water propeller characteristics/1 -> Mux/1, Product/2
  uvw/1 -> Selector/1
  Selector/1 -> Product1/2
  Mux/1 -> prop_tau/1

== system hydrofoil_sim_unified/Hydrofoil Craft/Pulse ==
  in : Inport
  Add{1..4} (4 alike) : Sum
  Demux : Demux  Outputs=6
  Mux : Mux  Inputs=6
  Ramp : simulink/Sources/Ramp  slope=800  start=4  InitialOutput=0
  Ramp1 : simulink/Sources/Ramp  slope=-800  start=4.5  InitialOutput=0
  Ramp2 : simulink/Sources/Ramp  slope=-800  start=5  InitialOutput=0
  Ramp3 : simulink/Sources/Ramp  slope=800  start=5.5  InitialOutput=0
  Scope : Scope
  Step1 : Step  Time=4.5  After=500  SampleTime=0
  Step2 : Step  Time=5.5  After=-500  SampleTime=0
  Sum1 : Sum  Inputs=|++
  out : Outport
  wires:
  in/1 -> Demux/1
  Demux/1 -> Mux/1
  Demux/2 -> Mux/2
  Demux/3 -> Mux/3
  Demux/5 -> Mux/5
  Demux/6 -> Mux/6
  Mux/1 -> out/1
  Sum1/1 -> Mux/4
  Demux/4 -> Sum1/1
  Add2/1 -> Add4/1
  Add3/1 -> Add4/2
  Ramp/1 -> Add2/1
  Ramp1/1 -> Add2/2
  Ramp2/1 -> Add3/1
  Ramp3/1 -> Add3/2
  Add4/1 -> Sum1/2, Scope/1

== system hydrofoil_sim_unified/sense/GPS ==
  uvw : Inport
  euler_angle : Inport  Port=2
  BF2NED : mssSimulink/Modelling/Kinematics/Euler angles to rotation matrix
  Product : Product  Multiplication=Matrix(*)
  Selector : Selector  InputPortWidth=3  IndexOptions=Index vector (dialog)  Indices=[1]  OutputSizes=1
  Sum : Sum  Inputs=|++
  Zero-Order Hold : ZeroOrderHold  SampleTime=1/10
  gps_noise : RandomNumber  Variance=var_gps  Seed=seed_gps  SampleTime=1/200
  V_gps : Outport
  wires:
  euler_angle/1 -> BF2NED/1
  BF2NED/1 -> Product/1
  uvw/1 -> Product/2
  Product/1 -> Selector/1
  Selector/1 -> Sum/1
  gps_noise/1 -> Sum/2
  Sum/1 -> Zero-Order Hold/1
  Zero-Order Hold/1 -> V_gps/1

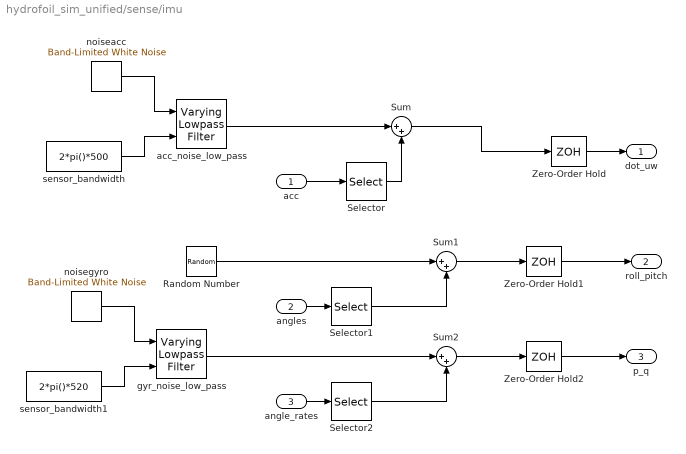
== system hydrofoil_sim_unified/sense/imu ==
  acc : Inport
  angles : Inport  Port=2
  angle_rates : Inport  Port=3
  Random Number : RandomNumber  Variance=[var_angle var_angle]  Seed=[seed_roll seed_pitch]  SampleTime=1/200
  Selector : Selector  InputPortWidth=3  IndexOptions=Index vector (dialog)  Indices=[1 3]  OutputSizes=1
  Selector1 : Selector  InputPortWidth=3  IndexOptions=Index vector (dialog)  Indices=[1 2]  OutputSizes=1
  Selector2 : Selector  InputPortWidth=3  IndexOptions=Index vector (dialog)  Indices=[1 2]  OutputSizes=1
  Sum : Sum  Inputs=|++
  Sum1 : Sum  Inputs=|++
  Sum2 : Sum  Inputs=|++
  Zero-Order Hold : ZeroOrderHold  SampleTime=1/100
  Zero-Order Hold1 : ZeroOrderHold  SampleTime=1/100
  Zero-Order Hold2 : ZeroOrderHold  SampleTime=1/100
  acc_noise_low_pass : cstblocks/Linear Parameter Varying/Varying Lowpass Filter  N=1
  gyr_noise_low_pass : cstblocks/Linear Parameter Varying/Varying Lowpass Filter  N=1
  noiseacc : simulink/Sources/Band-Limited White Noise  Cov=[psd_acc psd_acc]  Ts=1/2000  seed=[seed_accX seed_accZ]
  noisegyro : simulink/Sources/Band-Limited White Noise  Cov=[psd_gyro psd_gyro]  Ts=1/2000  seed=[seed_gyroX seed_gyroY]
  sensor_bandwidth : Constant  Value=2*pi()*500
  sensor_bandwidth1 : Constant  Value=2*pi()*520
  dot_uw : Outport
  roll_pitch : Outport  Port=2
  p_q : Outport  Port=3
  wires:
  Zero-Order Hold/1 -> dot_uw/1
  Sum/1 -> Zero-Order Hold/1
  acc/1 -> Selector/1
  Selector/1 -> Sum/2
  angles/1 -> Selector1/1
  angle_rates/1 -> Selector2/1
  Selector1/1 -> Sum1/2
  gyr_noise_low_pass/1 -> Sum2/1
  Selector2/1 -> Sum2/2
  Sum1/1 -> Zero-Order Hold1/1
  Zero-Order Hold1/1 -> roll_pitch/1
  Zero-Order Hold2/1 -> p_q/1
  Sum2/1 -> Zero-Order Hold2/1
  sensor_bandwidth/1 -> acc_noise_low_pass/2
  acc_noise_low_pass/1 -> Sum/1
  noiseacc/1 -> acc_noise_low_pass/1
  sensor_bandwidth1/1 -> gyr_noise_low_pass/2
  noisegyro/1 -> gyr_noise_low_pass/1
  Random Number/1 -> Sum1/1

== system hydrofoil_sim_unified/sense/sonar ==
  position : Inport
  theta : Inport  Port=2
  environment : Inport  Port=3
  angle_noise : Inport  Port=4
  BF2NED : mssSimulink/Modelling/Kinematics/Euler angles to rotation matrix
  Demux : Demux  Outputs=2
  Mux : Mux  Inputs=3
  Random Number : RandomNumber  Variance=var_sonar  Seed=seed_sonar  SampleTime=1/20
  Scope : Scope  NumInputPorts=2
  Selector : Selector  InputPortWidth=3  IndexOptions=Index vector (dialog)  Indices=[3]  OutputSizes=1
  Sum : Sum  Inputs=|++
  getCGheight : MATLAB Function  TreatAsAtomicUnit=on  SystemSampleTime=1/20
  sensor : Subsystem
  sonarpos : Constant  Value=sonar_position
  measured : Outport
  filtered : Outport  Port=2
  wires:
  sonarpos/1 -> getCGheight/3(sonar_position), sensor/4(sonar_pos)
  theta/1 -> sensor/3(angles)
  environment/1 -> sensor/1(environment)
  BF2NED/1 -> getCGheight/2(DCM)
  position/1 -> Selector/1, sensor/2(position)
  getCGheight/2(height_filtered) -> filtered/1
  Sum/1 -> getCGheight/1(h_s)
  sensor/1(sonar_height) -> Sum/2
  getCGheight/1(height_measured) -> Scope/1, measured/1
  angle_noise/1 -> Demux/1
  Demux/1 -> Mux/1
  Demux/2 -> Mux/2
  Selector/1 -> Scope/2
  Random Number/1 -> Sum/1
  Mux/1 -> BF2NED/1

== system hydrofoil_sim_unified/Controller [Variant]/LPV-MPC-IDP/Reference Previewer ==
  MATLAB Function : MATLAB Function  TreatAsAtomicUnit=on
  Memory1 : Memory  InheritSampleTime=on  LinearizeAsDelay=on
  sequence : Outport
  current : Outport  Port=2
  wires:
  MATLAB Function/1(seq) -> sequence/1
  MATLAB Function/2(first) -> current/1
  Memory1/1 -> MATLAB Function/1(t)
  MATLAB Function/3(next_t) -> Memory1/1

== system hydrofoil_sim_unified/Controller [Variant]/LPV-MPC-IP/Reference Previewer ==
  MATLAB Function : MATLAB Function  TreatAsAtomicUnit=on
  Memory1 : Memory  InheritSampleTime=on  LinearizeAsDelay=on
  sequence : Outport
  current : Outport  Port=2
  wires:
  MATLAB Function/1(seq) -> sequence/1
  MATLAB Function/2(first) -> current/1
  Memory1/1 -> MATLAB Function/1(t)
  MATLAB Function/3(next_t) -> Memory1/1

== system hydrofoil_sim_unified/Controller [Variant]/MPC-IDP/Reference Previewer ==
  MATLAB Function : MATLAB Function  TreatAsAtomicUnit=on
  Memory1 : Memory  InheritSampleTime=on  LinearizeAsDelay=on
  sequence : Outport
  current : Outport  Port=2
  wires:
  MATLAB Function/1(seq) -> sequence/1
  MATLAB Function/2(first) -> current/1
  Memory1/1 -> MATLAB Function/1(t)
  MATLAB Function/3(next_t) -> Memory1/1

== system hydrofoil_sim_unified/Controller [Variant]/MPC-IOP/Reference Previewer ==
  MATLAB Function : MATLAB Function  TreatAsAtomicUnit=on
  Memory1 : Memory  InheritSampleTime=on  LinearizeAsDelay=on
  sequence : Outport
  current : Outport  Port=2
  wires:
  MATLAB Function/1(seq) -> sequence/1
  MATLAB Function/2(first) -> current/1
  Memory1/1 -> MATLAB Function/1(t)
  MATLAB Function/3(next_t) -> Memory1/1

== system hydrofoil_sim_unified/Controller [Variant]/MPC-IP/Reference Previewer ==
  MATLAB Function : MATLAB Function  TreatAsAtomicUnit=on
  Memory1 : Memory  InheritSampleTime=on  LinearizeAsDelay=on
  sequence : Outport
  current : Outport  Port=2
  wires:
  MATLAB Function/1(seq) -> sequence/1
  MATLAB Function/2(first) -> current/1
  Memory1/1 -> MATLAB Function/1(t)
  MATLAB Function/3(next_t) -> Memory1/1
